simulink model "velocity_control_dc"  (R2022b)
settings: Solver=ode1  StartTime=0.0  StopTime=10.0  FixedStep=0.001  RelTol=1e-3
undefined symbols (not defined in the file): a, b, Ki, Kp
settings Model: Creator=sokse  LastModifiedBy=sokse

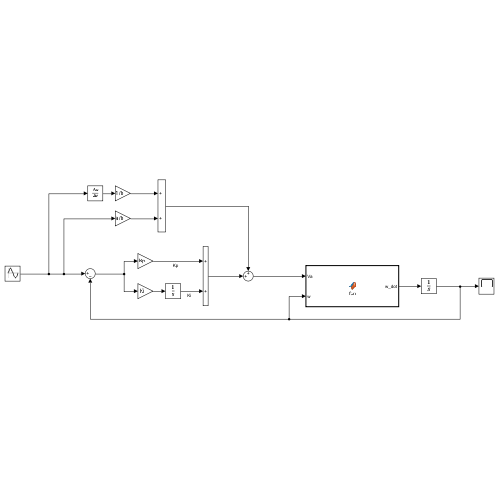
[thumbnail: Simulink's stored preview of the top-level diagram]
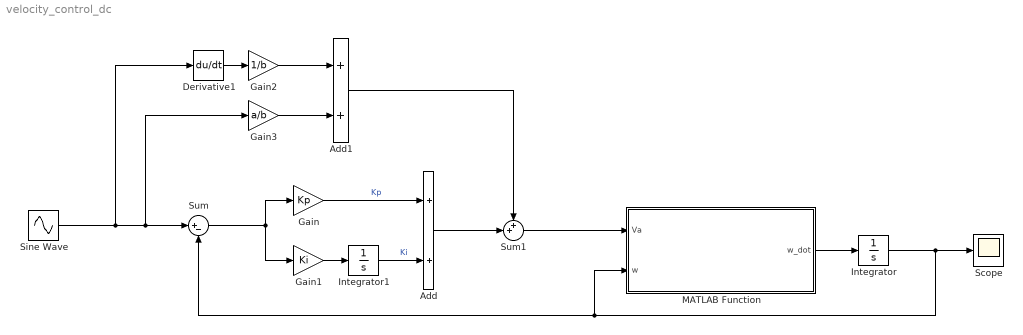
== system velocity_control_dc ==
  Add : Sum
  Add1 : Sum
  Derivative1 : Derivative
  Gain : Gain  Gain=Kp
  Gain1 : Gain  Gain=Ki
  Gain2 : Gain  Gain=1/b
  Gain3 : Gain  Gain=a/b
  Integrator : Integrator
  Integrator1 : Integrator
  MATLAB Function : MATLAB Function  TreatAsAtomicUnit=on
  Scope : Scope
  Sine Wave : Sin  Amplitude=10  Frequency=2*pi*4  SampleTime=0
  Sum : Sum  Inputs=|+-
  Sum1 : Sum  Inputs=++|
  wires:
  Sum1/1 -> MATLAB Function/1(Va)
  Gain1/1 -> Integrator1/1
  Sum/1 -> Gain1/1, Gain/1
  Add/1 -> Sum1/2
  Gain/1 -> Add/1  "Kp"
  MATLAB Function/1(w_dot) -> Integrator/1
  Integrator/1 -> Scope/1, MATLAB Function/2(w), Sum/2
  Integrator1/1 -> Add/2  "Ki"
  Derivative1/1 -> Gain2/1
  Sine Wave/1 -> Derivative1/1, Gain3/1, Sum/1
  Gain2/1 -> Add1/1
  Gain3/1 -> Add1/2
  Add1/1 -> Sum1/1

== matlab function velocity_control_dc/MATLAB Function ==
  data: Va input; w_dot output; w input
function w_dot = fcn(Va,w)

a = 10; 
b = 25; 
w_dot = -a*w+b*Va;
